simulink model "obs_det"  (R2022b)
settings: Solver=FixedStepDiscrete  StartTime=0.0  StopTime=10.0  FixedStep=0.01  RelTol=1e-3
libraries: mobileRoboticsTrainingLib x5
settings Model: Creator=Asitha  LastModifiedBy=Asitha

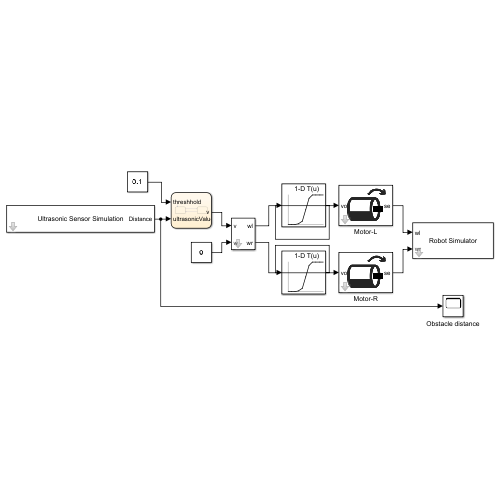
[thumbnail: Simulink's stored preview of the top-level diagram]
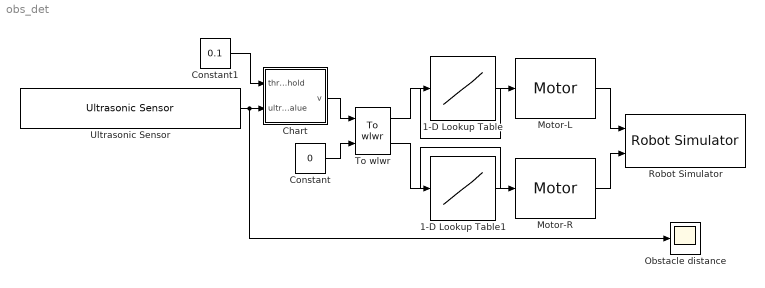
== system obs_det ==
  1-D Lookup Table : Lookup_n-D  NumberOfTableDimensions=1  BreakpointsForDimension1=[-5:5]  Table=tanh([-5:5])  InternalRulePriority=Speed  RndMeth=Simplest
  1-D Lookup Table1 : Lookup_n-D  NumberOfTableDimensions=1  BreakpointsForDimension1=[-5:5]  Table=tanh([-5:5])  InternalRulePriority=Speed  RndMeth=Simplest
  Chart : Stateflow chart  TreatAsAtomicUnit=on
  Constant : Constant  Value=0
  Constant1 : Constant  Value=0.1
  Motor-L : mobileRoboticsTrainingLib/Motor  motorPlant=1  sensorType=Speed
      settings: SourceProductName=Mobile Robotics Training Library
  Motor-R : mobileRoboticsTrainingLib/Motor  motorPlant=1  sensorType=Speed
      settings: SourceProductName=Mobile Robotics Training Library
  Obstacle distance : Scope
  Robot Simulator : mobileRoboticsTrainingLib/Robot Simulator  Priority=99  mapVar=mapForSim  startX=3.743  startY=1.1565  startTheta=90  axleLength=0.1  wheelR=0.05
      link override Soft Real Time: x=1
  To wlwr : mobileRoboticsTrainingLib/To wlwr  axleLength=0.1  wheelR=0.05
  Ultrasonic Sensor : mobileRoboticsTrainingLib/Ultrasonic Sensor  mapVar=mapForSim  maxSenRange=2  minSenRange=0.02  senRes=0.01  sensOff=[0 0]
      settings: SourceProductName=Mobile Robotics Training Library
  wires:
  Ultrasonic Sensor/1 -> Chart/2(ultrasonicValue), Obstacle distance/1
  Constant/1 -> To wlwr/2
  To wlwr/1 -> 1-D Lookup Table/1
  To wlwr/2 -> 1-D Lookup Table1/1
  1-D Lookup Table/1 -> Motor-L/1
  1-D Lookup Table1/1 -> Motor-R/1
  Motor-L/1 -> Robot Simulator/1
  Motor-R/1 -> Robot Simulator/2
  Constant1/1 -> Chart/1(threshhold)
  Chart/1(v) -> To wlwr/1

== stateflow chart obs_det/Chart ==
  state GoForward
    v = 0.1
  state Stop
    v = 0
  (default) -> GoForward
  GoForward -> Stop : [ultrasonicValue <=threshhold]
  Stop -> GoForward : [ultrasonicValue > threshhold]
  data: threshhold input; ultrasonicValue input; v output
